simulink model "embedded_with_delay"  (Simulink 7.1)
settings: Solver=ode45  StartTime=0.0  StopTime=10.0  RelTol=1e-3
settings Model: Creator=Administrator  LastModifiedBy=Administrator

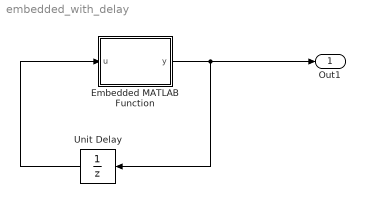
== system embedded_with_delay ==
  Embedded MATLAB Function : Stateflow chart
  Unit Delay : UnitDelay  Orientation=left
  Out1 : Outport  PortDimensions=[3]  DataType=single  OutDataType=sfix(16)  OutScaling=2^0  OutDataTypeStr=single
  wires:
  Embedded MATLAB Function/1(y) -> Unit Delay/1, Out1/1
  Unit Delay/1 -> Embedded MATLAB Function/1(u)

== matlab function Embedded MATLAB Function ==
  data: u input single size=[3]; y output single size=[3]
function y = fcn(u)
% This block supports the Embedded MATLAB subset.
% See the help menu for details. 

y = u;
